simulink model "ThreeDOF_Rocket_Simulator_v6_MERGE"  (R2024a)
settings: Solver=VariableStepAuto  StartTime=0.0  StopTime=30  RelTol=1e-3
libraries: shared3dof x1, simulink_extras x1, simulink x1
settings Model: Creator=giuse  LastModifiedBy=giuse
settings OptimizationCC: ReuseModelBlockBuffer=off
settings DebuggingCC: UnconnectedInputMsg=warning  UnconnectedOutputMsg=warning  UnconnectedLineMsg=warning
settings ModelReferenceCC: EnableRefExpFcnMdlSchedulingChecks=on
settings RTWCC: GPUComputeCapability=3.5  DLArmComputeVersion=19.05

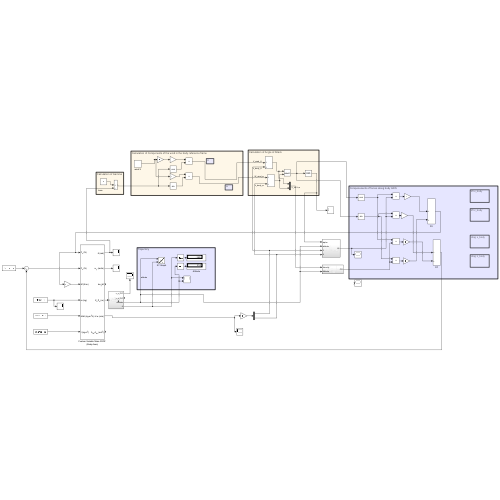
[thumbnail: Simulink's stored preview of the top-level diagram]
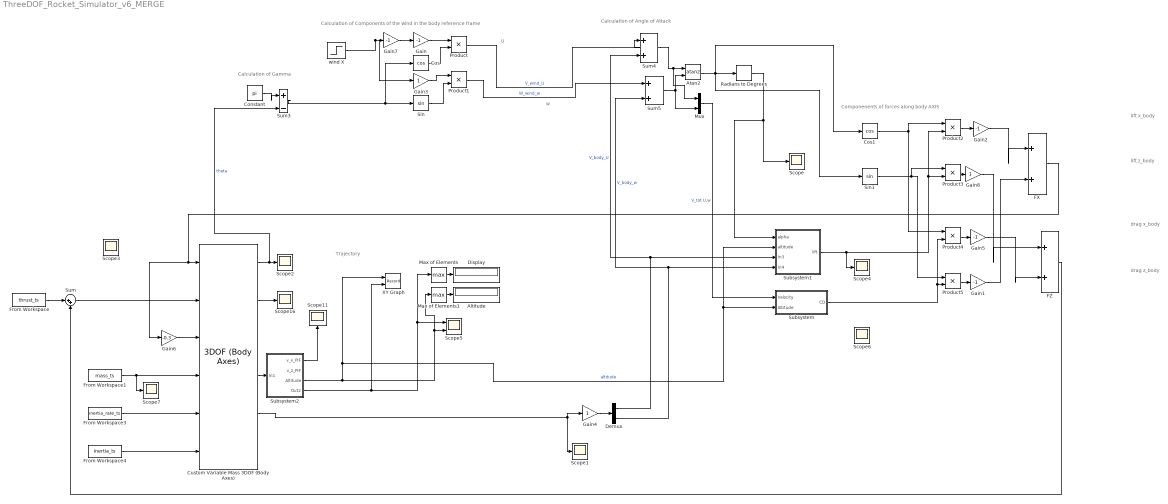
== system ThreeDOF_Rocket_Simulator_v6_MERGE ==
  note: lift x_body
  note: Componenents of forces along body AXIS
  note: Calculation of Angle of Attack
  note: U
  note: Calculation of Components of the wind in the body reference frame
  note: Calculation of Gamma
  note: Trajectory
  note: w
  note: lift z_body
  note: drag z_body
  note: drag x_body
  Altitude : Display
  Atan2 : Trigonometry  Operator=atan2
  Constant : Constant  Value=pi
  Cos : Trigonometry  Operator=cos
  Cos1 : Trigonometry  Operator=cos
  Custom Variable Mass 3DOF (Body Axes) : shared3dof/3DOF (Body Axes)  units=Metric (MKS)  mtype=Custom Variable  v_ini=0  theta_ini=pi  alpha_ini=pi/2  pos_ini=[0 0]  q_ini=0  mass=1.0  mass_e=0.5  mass_f=3.0  Iyy=1.0  Iyy_e=0.5  Iyy_f=3.0  g_in=Internal  g=9.81  vre_flag=off  abi_flag=off  aMode=0  vel_statename=''  theta_statename=''  pos_statename=''  q_statename=''  mass_statename=''
  Demux : Demux  Outputs=2
  Display : Display
  FX : Sum  Inputs=|++
  FZ : Sum  Inputs=|++
  From Workspace : FromWorkspace  VariableName=thrust_ts
  From Workspace1 : FromWorkspace  VariableName=mass_ts
  From Workspace3 : FromWorkspace  VariableName=inertia_rate_ts
  From Workspace4 : FromWorkspace  VariableName=inertia_ts
  Gain{,1..2,5,7} (5 alike) : Gain  Gain=-1
  Gain3 : Gain
  Gain4 : Gain
  Gain6 : Gain  Gain=-0.3
  Gain8 : Gain
  Max of Elements : MinMax  Function=max
  Max of Elements1 : MinMax  Function=max
  Mux : Mux  Inputs=2
  Product{,1..5} (6 alike) : Product
  Radians to Degrees : simulink_extras/Transformations/Radians to Degrees
  Scope{,1..4,6..7,11,16} (9 alike) : Scope
  Scope5 : Scope  NumInputPorts=2
  Sin : Trigonometry
  Sin1 : Trigonometry
  Subsystem : Subsystem
  Subsystem1 : Subsystem
  Subsystem2 : Subsystem
  Sum : Sum  Inputs=|++
  Sum3 : Sum  Inputs=|+-
  Sum4 : Sum  Inputs=|++
  Sum5 : Sum
  XY Graph : Record  FileSettingsInternal="{\"entries\":[{\"content\":{\"excelSettings\":{\"content\":{},\"type\":\"Streamout.ExcelSettings\"}},\"type\":\"Streamout.FileSettingStorage\",\"uuid\":\"\"}],\"packageUris\":[\"http:\\/\\/schema.mathworks.com\\/mf0\\/streamout_blocks\\/R2020a\"],\"version\":\"1.0\"}"  Layout=[1 1]  SignalsInternal="{\"entries\":[{\"content\":{\"signals\":[{\"content\":{\"blockPath\":[],\"dimensions\":[1],\"domain\":\"\",\"lineColor\":\"#64d413\",\"plots\":[ 1 ],\"port\":1,\"sid\":[\"\"],\"signalID\":1,\"signalName\":\"altitude\"},\"type\":\"RecordBlkView.Signal\",\"uuid\":\"\"},{\"content\":{\"blockPath\":[],\"dimensions\":[1],\"domain\":\"\",\"lineColor\":\"#ff13a6\",\"plots\":[ 1 ],\"port\":2,\"sid\":[\"\"],\"signalID\":2,\"signalName\":\"Subsystem2:4\"},\"type\":\"RecordBlkView.Signal\",\"uuid\":\"\"}]},\"type\":\"RecordBlkView.InputSignals\",\"uuid\":\"\"}],\"packageUris\":[\"http:\\/\\/schema.mathworks.com\\/mf0\\/streamout_blocks\\/R2020a\"],\"version\":\"1.0\"}"  VisualizationBindings="{\"xyplotplugin\":{\"info\":[{\"series\":[{\"bindingParametersList\":[{\"parameter\":\"X-Axis\",\"signalID\":2,\"signalName\":\"Subsystem2:4\"},{\"parameter\":\"Y-Axis\",\"signalID\":1,\"signalName\":\"altitude\"}],\"seriesID\":0}],\"subplotID\":1}]}}"  CompatibilityTag=XY
  wind X : Step  Time=0.351  After=2  SampleTime=0
  wires:
  From Workspace1/1 -> Scope7/1, Custom Variable Mass 3DOF (Body Axes)/4
  From Workspace4/1 -> Custom Variable Mass 3DOF (Body Axes)/6
  From Workspace/1 -> Sum/1
  Sum/1 -> Custom Variable Mass 3DOF (Body Axes)/2
  Custom Variable Mass 3DOF (Body Axes)/4 -> Subsystem2/1(In1)
  Custom Variable Mass 3DOF (Body Axes)/5 -> Scope1/1, Gain4/1
  Subsystem2/3(Altitude) -> Subsystem1/2(altitude), Subsystem/2(Altitude), XY Graph/1, Max of Elements1/1, Scope5/2  "altitude"
  Subsystem2/4(Out2) -> Max of Elements/1, Scope5/1, XY Graph/2
  Max of Elements/1 -> Display/1
  Max of Elements1/1 -> Altitude/1
  Custom Variable Mass 3DOF (Body Axes)/1 -> Sum3/2, Scope2/1  "theta"
  Demux/2 -> Sum5/2, Subsystem1/4(In4)  "V_body_w"
  Subsystem2/1(v_x_PIF) -> Scope11/1
  Demux/1 -> Subsystem1/3(In3), Sum4/2  "V_body_U"
  Custom Variable Mass 3DOF (Body Axes)/2 -> Scope16/1
  From Workspace3/1 -> Custom Variable Mass 3DOF (Body Axes)/5
  Constant/1 -> Sum3/1
  Gain/1 -> Product/1
  Cos/1 -> Product/2
  Sum3/1 -> Sin/1, Cos/1
  Gain3/1 -> Product1/1
  Sin/1 -> Product1/2
  Product/1 -> Sum4/1  "V_wind_U"
  Product1/1 -> Sum5/1  "W_wind_w"
  Atan2/1 -> Radians to Degrees/1, Cos1/1, Sin1/1
  Cos1/1 -> Product4/1, Product2/1
  Sin1/1 -> Product5/1, Product3/1
  Subsystem1/1(lift) -> Scope4/1, Product2/2, Product3/2
  Product5/1 -> Gain1/1
  Product2/1 -> Gain2/1
  Gain2/1 -> FX/1
  Gain1/1 -> FX/2
  Gain6/1 -> Custom Variable Mass 3DOF (Body Axes)/3
  Product4/1 -> Gain5/1
  Gain5/1 -> FZ/2
  Radians to Degrees/1 -> Scope/1, Subsystem1/1(alpha)
  FZ/1 -> Sum/2
  Gain4/1 -> Demux/1
  Sum4/1 -> Mux/1, Atan2/1
  Sum5/1 -> Mux/2, Atan2/2
  wind X/1 -> Gain3/1, Gain7/1
  Gain7/1 -> Gain/1
  Mux/1 -> Subsystem/1(Velocity)  "V_tot U,w"
  Product3/1 -> Gain8/1
  Gain8/1 -> FZ/1
  FX/1 -> Gain6/1, Custom Variable Mass 3DOF (Body Axes)/1
  Subsystem/1(CD) -> Product4/2, Product5/2

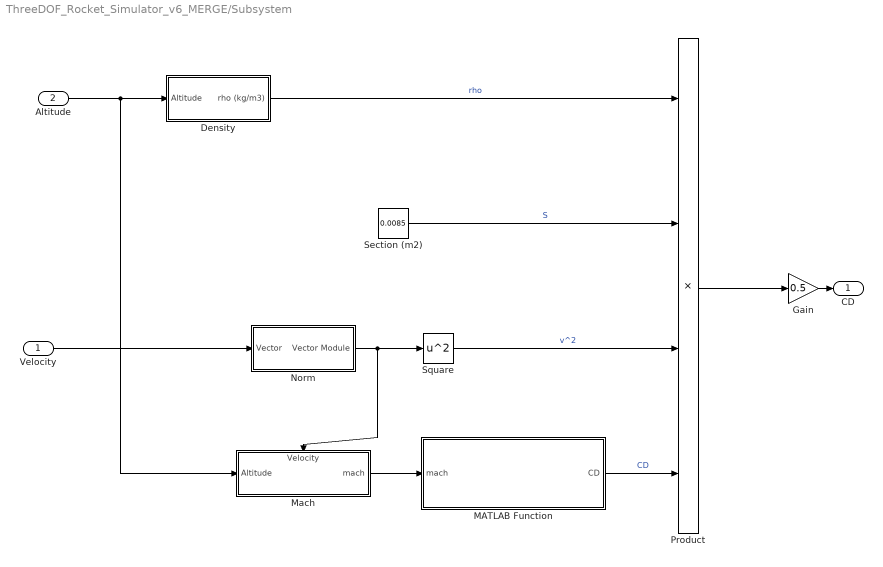
== system ThreeDOF_Rocket_Simulator_v6_MERGE/Subsystem ==
  Velocity : Inport
  Altitude : Inport  Port=2
  Density : Subsystem
  Gain : Gain  Gain=0.5
  MATLAB Function : MATLAB Function  TreatAsAtomicUnit=on
  Mach : Subsystem
      settings: PortSchema="{\"entries\":[{\"content\":{\"sides\":[{\"content\":{\"connectorIds\":[\"In1\"]},\"type\":\"ConnectorPlacement.EquallySpacedRectSide\",\"uuid\":\"3d39723d-d359-4481-8e57-a1560243478f\"},{\"content\":{\"connectorIds\":[\"Out1\"],\"side\":\"RIGHT\"},\"type\":\"ConnectorPlacement.EquallySpacedRectSide\",\"uuid\":\"25d074cf-118b-4153-b466-e753361fe918\"},{\"content\":{\"connectorIds\":[\"In2\"],\"side\":\"TOP\"},\"type\":\"ConnectorPlacement.EquallySpacedRectSide\",\"uuid\":\"b814a212-e79e-4e83-ade8-85d301fd4927\"}]},\"type\":\"ConnectorPlacement.EquallySpacedConnector\",\"uuid\":\"c89f41df-1f7d-46ca-b296-160aff391222\"}],\"packageUris\":[\"http://schema.mathworks.com/mf0/Connector/R2020b\"],\"version\":\"1.0\"}"
  Norm : Subsystem
  Product : Product  Inputs=4
  Section (m2) : Constant  Value=0.0085
  Square : Math  Operator=square
  CD : Outport
  wires:
  Density/1(rho (kg/m3)) -> Product/1  "rho"
  Square/1 -> Product/3  "v^2"
  Velocity/1 -> Norm/1(Vector)
  Altitude/1 -> Mach/1(Altitude), Density/1(Altitude)
  Mach/1(mach) -> MATLAB Function/1(mach)
  MATLAB Function/1(CD) -> Product/4  "CD"
  Norm/1(Vector Module) -> Square/1, Mach/2(Velocity)
  Section (m2)/1 -> Product/2  "S"
  Product/1 -> Gain/1
  Gain/1 -> CD/1

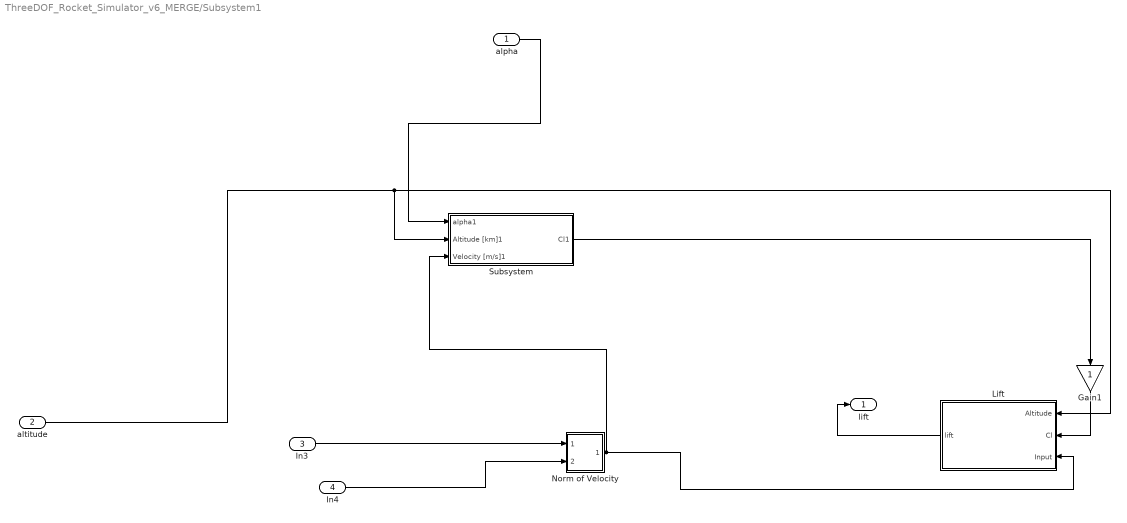
== system ThreeDOF_Rocket_Simulator_v6_MERGE/Subsystem1 ==
  alpha : Inport
  altitude : Inport  Port=2
  In3 : Inport  Port=3
  In4 : Inport  Port=4
  Gain1 : Gain
  Lift : Subsystem
  Norm of Velocity : Subsystem
  Subsystem : Subsystem
  lift : Outport
  wires:
  Norm of Velocity/1(Input) -> Subsystem/3(Velocity [m/s]1), Lift/3(Input)
  Lift/1(lift) -> lift/1
  Gain1/1 -> Lift/2(Cl)
  altitude/1 -> Subsystem/2(Altitude [km]1), Lift/1(Altitude)
  In4/1 -> Norm of Velocity/2(In2)
  In3/1 -> Norm of Velocity/1(In1)
  alpha/1 -> Subsystem/1(alpha1)
  Subsystem/1(Cl1) -> Gain1/1

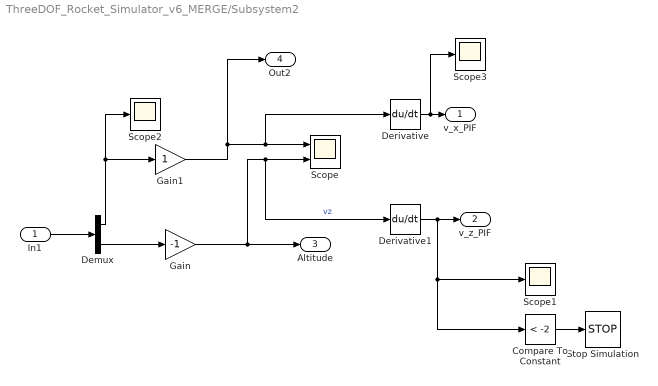
== system ThreeDOF_Rocket_Simulator_v6_MERGE/Subsystem2 ==
  In1 : Inport
  Compare To Constant : simulink/Logic and Bit Operations/Compare To Constant  relop=<  const=-2  OutDataTypeStr=boolean
  Demux : Demux  Outputs=2
  Derivative : Derivative
  Derivative1 : Derivative
  Gain : Gain  Gain=-1
  Gain1 : Gain
  Scope : Scope  NumInputPorts=2
  Scope1 : Scope
  Scope2 : Scope
  Scope3 : Scope
  Stop Simulation : Stop
  v_x_PIF : Outport
  v_z_PIF : Outport  Port=2
  Altitude : Outport  Port=3
  Out2 : Outport  Port=4
  wires:
  Demux/2 -> Gain/1
  Gain/1 -> Altitude/1, Derivative1/1, Scope/2  "vz"
  In1/1 -> Demux/1
  Demux/1 -> Scope2/1, Gain1/1
  Gain1/1 -> Out2/1, Derivative/1, Scope/1
  Derivative1/1 -> Compare To Constant/1, Scope1/1, v_z_PIF/1
  Compare To Constant/1 -> Stop Simulation/1
  Derivative/1 -> Scope3/1, v_x_PIF/1

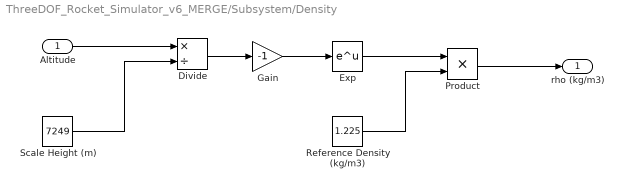
== system ThreeDOF_Rocket_Simulator_v6_MERGE/Subsystem/Density ==
  Altitude : Inport
  Divide : Product  Inputs=*/
  Exp : Math
  Gain : Gain  Gain=-1
  Product : Product
  Reference Density (kg/m3) : Constant  Value=1.225
  Scale Height (m) : Constant  Value=7249
  rho (kg/m3) : Outport
  wires:
  Altitude/1 -> Divide/1
  Scale Height (m)/1 -> Divide/2
  Divide/1 -> Gain/1
  Gain/1 -> Exp/1
  Exp/1 -> Product/1
  Reference Density (kg/m3)/1 -> Product/2
  Product/1 -> rho (kg/m3)/1

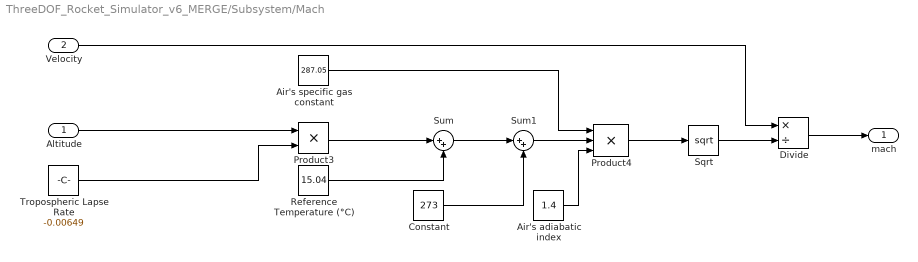
== system ThreeDOF_Rocket_Simulator_v6_MERGE/Subsystem/Mach ==
  Altitude : Inport
  Velocity : Inport  Port=2
  Air's adiabatic index : Constant  Value=1.4
  Air's specific gas constant : Constant  Value=287.05
  Constant : Constant  Value=273
  Divide : Product  Inputs=*/
  Product3 : Product
  Product4 : Product  Inputs=3
  Reference Temperature (°C) : Constant  Value=15.04
  Sqrt : Sqrt
  Sum : Sum  Inputs=|++
  Sum1 : Sum  Inputs=|++
  Tropospheric Lapse Rate : Constant  Value=-0.00649
  mach : Outport
  wires:
  Product4/1 -> Sqrt/1
  Product3/1 -> Sum/1
  Air's adiabatic index/1 -> Product4/3
  Tropospheric Lapse Rate/1 -> Product3/2
  Air's specific gas constant/1 -> Product4/1
  Sum/1 -> Sum1/1
  Reference Temperature (°C)/1 -> Sum/2
  Altitude/1 -> Product3/1
  Velocity/1 -> Divide/1
  Divide/1 -> mach/1
  Constant/1 -> Sum1/2
  Sum1/1 -> Product4/2
  Sqrt/1 -> Divide/2

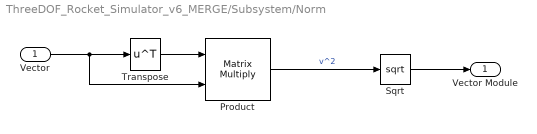
== system ThreeDOF_Rocket_Simulator_v6_MERGE/Subsystem/Norm ==
  Vector : Inport
  Product : Product  Multiplication=Matrix(*)
  Sqrt : Sqrt
  Transpose : Math  Operator=transpose
  Vector Module : Outport
  wires:
  Vector/1 -> Product/2, Transpose/1
  Product/1 -> Sqrt/1  "v^2"
  Sqrt/1 -> Vector Module/1
  Transpose/1 -> Product/1

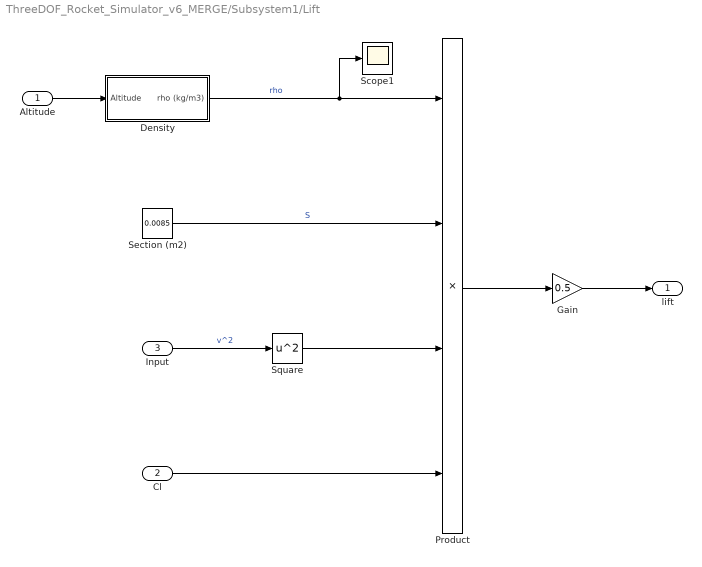
== system ThreeDOF_Rocket_Simulator_v6_MERGE/Subsystem1/Lift ==
  Altitude : Inport
  Cl : Inport  Port=2
  Input : Inport  Port=3
  Density : Subsystem
  Gain : Gain  Gain=0.5
  Product : Product  Inputs=4
  Scope1 : Scope
  Section (m2) : Constant  Value=0.0085
  Square : Math  Operator=square
  lift : Outport
  wires:
  Altitude/1 -> Density/1(Altitude)
  Density/1(rho (kg/m3)) -> Scope1/1, Product/1  "rho"
  Section (m2)/1 -> Product/2  "S"
  Product/1 -> Gain/1
  Cl/1 -> Product/4
  Input/1 -> Square/1  "v^2"
  Square/1 -> Product/3
  Gain/1 -> lift/1

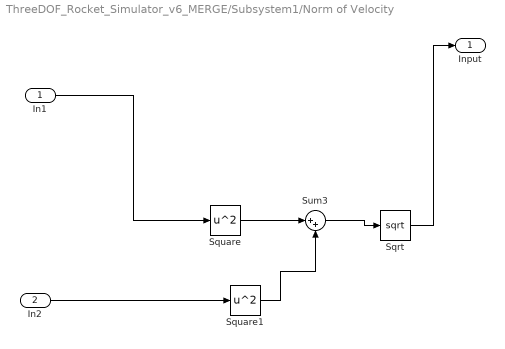
== system ThreeDOF_Rocket_Simulator_v6_MERGE/Subsystem1/Norm of Velocity ==
  In1 : Inport
  In2 : Inport  Port=2
  Sqrt : Sqrt
  Square : Math  Operator=square
  Square1 : Math  Operator=square
  Sum3 : Sum  Inputs=|++
  Input : Outport
  wires:
  Square1/1 -> Sum3/2
  Sqrt/1 -> Input/1
  Square/1 -> Sum3/1
  Sum3/1 -> Sqrt/1
  In2/1 -> Square1/1
  In1/1 -> Square/1

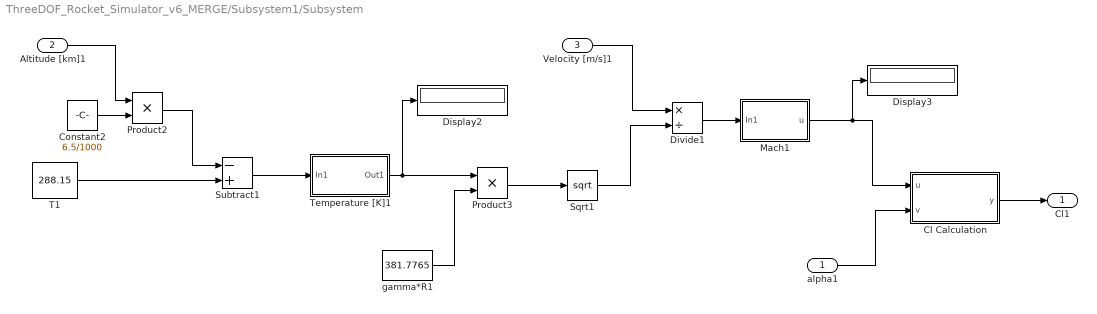
== system ThreeDOF_Rocket_Simulator_v6_MERGE/Subsystem1/Subsystem ==
  alpha1 : Inport
  Altitude [km]1 : Inport  Port=2
  Velocity [m/s]1 : Inport  Port=3
  Cl Calculation : MATLAB Function  TreatAsAtomicUnit=on
  Constant2 : Constant  Value=6.5/1000
  Display2 : Display
  Display3 : Display
  Divide1 : Product  Inputs=*/
  Mach1 : Subsystem
  Product2 : Product
  Product3 : Product
  Sqrt1 : Sqrt
  Subtract1 : Sum  Inputs=-+
  T1 : Constant  Value=288.15
  Temperature [K]1 : Subsystem
  gamma*R1 : Constant  Value=381.7765
  Cl1 : Outport
  wires:
  Altitude [km]1/1 -> Product2/1
  Mach1/1(u) -> Display3/1, Cl Calculation/1(u)
  Product2/1 -> Subtract1/1
  Temperature [K]1/1(Out1) -> Display2/1, Product3/1
  Constant2/1 -> Product2/2
  Cl Calculation/1(y) -> Cl1/1
  gamma*R1/1 -> Product3/2
  Product3/1 -> Sqrt1/1
  alpha1/1 -> Cl Calculation/2(v)
  Velocity [m/s]1/1 -> Divide1/1
  Subtract1/1 -> Temperature [K]1/1(In1)
  Divide1/1 -> Mach1/1(In1)
  Sqrt1/1 -> Divide1/2
  T1/1 -> Subtract1/2

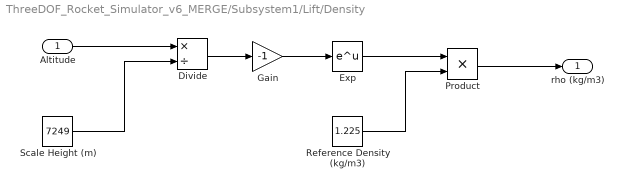
== system ThreeDOF_Rocket_Simulator_v6_MERGE/Subsystem1/Lift/Density ==
  Altitude : Inport
  Divide : Product  Inputs=*/
  Exp : Math
  Gain : Gain  Gain=-1
  Product : Product
  Reference Density (kg/m3) : Constant  Value=1.225
  Scale Height (m) : Constant  Value=7249
  rho (kg/m3) : Outport
  wires:
  Altitude/1 -> Divide/1
  Scale Height (m)/1 -> Divide/2
  Divide/1 -> Gain/1
  Gain/1 -> Exp/1
  Exp/1 -> Product/1
  Reference Density (kg/m3)/1 -> Product/2
  Product/1 -> rho (kg/m3)/1

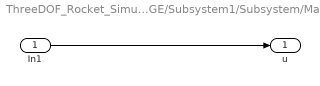
== system ThreeDOF_Rocket_Simulator_v6_MERGE/Subsystem1/Subsystem/Mach1 ==
  In1 : Inport
  u : Outport
  wires:
  In1/1 -> u/1

== system ThreeDOF_Rocket_Simulator_v6_MERGE/Subsystem1/Subsystem/Temperature [K]1 ==
  In1 : Inport
  Out1 : Outport
  wires:
  In1/1 -> Out1/1

== matlab function ThreeDOF_Rocket_Simulator_v6_MERGE/Subsystem/MATLAB Function ==
  data: CD output; mach input
function CD = mach_interp(mach)
cd_table = [0,0
0.001000 1.046000
0.003000 0.761000
0.006000 0.683000
0.009000 0.643000
0.013000 0.616000
0.016000 0.596000
0.019000 0.581000
0.022000 0.569000
0.025000 0.559000
0.028000 0.551000
0.031000 0.544000
0.034000 0.538000
0.038000 0.534000
0.041000 0.532000
0.044000 0.530000
0.047000 0.528000
0.050000 0.527000
0.053000 0.525000
0.056000 0.524000
0.059000 0.523000
0.063000 0.521000
0.066000 0.520000
0.069000 0.519000
0.072000 0.518000
0.075000 0.517000
0.078000 0.516000
0.081000 0.515000
0.085000 0.515000
0.088000 0.514000
0.091000 0.513000
0.094000 0.513000
0.097000 0.512000
0.100000 0.511000
0.103000 0.511000
0.107000 0.510000
0.111000 0.509000
0.119000 0.508000
0.129000 0.508000
0.145000 0.509000
0.161000 0.509000
0.177000 0.510000
0.193000 0.511000
0.209000 0.512000
0.226000 0.513000
0.242000 0.514000
0.258000 0.515000
0.275000 0.516000
0.292000 0.517000
0.309000 0.518000
0.326000 0.520000
0.343000 0.521000
0.361000 0.523000
0.378000 0.524000
0.396000 0.526000
0.413000 0.528000
0.431000 0.530000
0.448000 0.532000
0.466000 0.534000
0.483000 0.536000
0.500000 0.538000
0.517000 0.540000
0.533000 0.542000
0.550000 0.545000
0.566000 0.547000
0.583000 0.550000
0.599000 0.552000
0.615000 0.555000
0.631000 0.557000
0.646000 0.560000
0.662000 0.562000
0.677000 0.565000
0.692000 0.568000
0.708000 0.570000
0.722000 0.573000
0.737000 0.576000
0.752000 0.579000
0.766000 0.581000
0.780000 0.584000
0.794000 0.587000
0.808000 0.590000
0.821000 0.593000
0.835000 0.596000
0.848000 0.598000
0.861000 0.601000
0.874000 0.604000
0.887000 0.607000
0.899000 0.610000
0.911000 0.612000
0.920000 0.614000
0.925000 0.615000
0.926000 0.615000];
CD = spline(cd_table(:,1),cd_table(:,2),mach);

== matlab function ThreeDOF_Rocket_Simulator_v6_MERGE/Subsystem1/Subsystem/Cl Calculation ==
  data: u input; y output; v input
function y = fcn(u,v)

if u<1
% SUBSONIC CASE (linearized theory for a thin plate)
    y = ((2*pi*(v*2*pi)/360)./(sqrt(1-u.^2)))*13500/(2*pi*(52)^2).*2;

else
% SUPERSONIC CASE (interpolation)
    Cl_Dat1 = [0 0.6615 1.427]; % M = 0.5
    Cl_Dat2 = [0 0.8 1.688]; % M = 1
    Cl_Dat3 = [0 0.6265 1.322]; % M = 1.5
    Cl_Dat4 = [0 0.5565 1.186]; % M = 2

    % if the geometry of the rocket changes, 4 new simulations must be 
    % carried out for 3 alpha values (0 alpha/2 alpha)

    CL = [Cl_Dat1;Cl_Dat2;Cl_Dat3;Cl_Dat4];

    X = [0 2.5 5;0 2.5 5;0 2.5 5;0 2.5 5]; % alpha values ​​per column (simulations)
    Y = [0.5 0.5 0.5;1 1 1;1.5 1.5 1.5;2 2 2]; % Mach values per row (simulations)
    y = interp2(X,Y,CL,v,u);

end
